simulink model "Brk"  (R2016b)
settings: Solver=VariableStepAuto  StartTime=0.0  StopTime=10.0  RelTol=1e-3
settings Model: Creator=jiakui  LastModifiedBy=jiakui

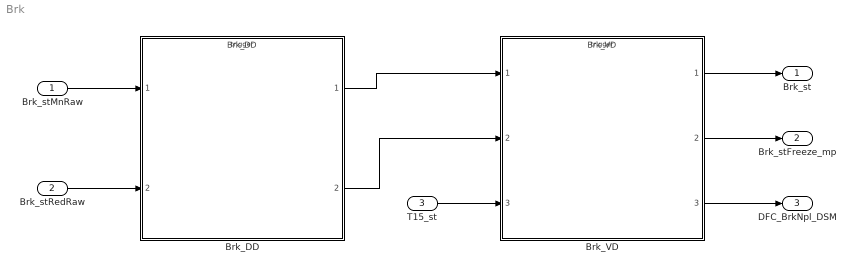
== system Brk ==
  Brk_stMnRaw : Inport  Description=State main brake switch, raw value  OutMin=0  OutMax=1  OutDataTypeStr=boolean
  Brk_stRedRaw : Inport  Description=State redundant brake switch, raw value  Port=2  OutMin=0  OutMax=1  OutDataTypeStr=boolean
  T15_st : Inport  Description=Terminal 15 status after debouncing  Port=3  OutDataTypeStr=Enum: Switch_conv
  Brk_DD : ModelReference  ModelNameDialog=Brk_DD  SimulationMode=Normal  ModelReferenceVersion=1.6  TriggerPortName=function  TriggerPortTriggerType=function-call  TriggerPortStatesWhenEnabling=held
  Brk_VD : ModelReference  ModelNameDialog=Brk_VD  SimulationMode=Normal  ModelReferenceVersion=1.10  TriggerPortName=function  TriggerPortTriggerType=function-call  TriggerPortStatesWhenEnabling=held
  Brk_st : Outport  Description=Brake switch state  OutMin=0  OutMax=255  OutDataTypeStr=State_uint8
  Brk_stFreeze_mp : Outport  Description=Measuring Point to indicate whether the brake plausibility state machine is in Neutral State  Port=2  OutMin=0  OutMax=1  OutDataTypeStr=boolean
  DFC_BrkNpl_DSM : Outport  Description="state of error\"DFC_BrkNpl\""  Port=3  OutMin=0  OutMax=1  OutDataTypeStr=boolean
  wires:
  Brk_stMnRaw/1 -> Brk_DD/1
  Brk_stRedRaw/1 -> Brk_DD/2
  Brk_DD/1 -> Brk_VD/1
  Brk_DD/2 -> Brk_VD/2
  T15_st/1 -> Brk_VD/3
  Brk_VD/1 -> Brk_st/1
  Brk_VD/2 -> Brk_stFreeze_mp/1
  Brk_VD/3 -> DFC_BrkNpl_DSM/1
